simulink model "gps_casestudy_1_16"  (R2023a)
settings: Solver=VariableStepAuto  StartTime=0.0  StopTime=10.0  RelTol=1e-3
settings Model: PacingRate=0.890000  ExtModeTrigDuration=100  Creator=simon  LastModifiedBy=simon
settings DataIOCC: StateSaveName=tmp_raccel_xout  OutputSaveName=tmp_raccel_yout1  SignalLoggingName=tmp_raccel_logsout
settings OptimizationCC: EfficientMapNaN2IntZero=off  AccelVerboseBuild=on
settings HardwareCC: TargetBitPerPointer=64  TargetBitPerSizeT=64  TargetBitPerPtrDiffT=64  TargetLongLongMode=on  TargetIntDivRoundTo=Zero  TargetEndianess=LittleEndian  TargetWordSize=64  TargetHWDeviceType=MATLAB Host  ProdEqTarget=off
settings RTWCC: SystemTargetFile=raccel.tlc  TemplateMakefile=raccel_default_tmf  RTWVerbose=off  RTWUseSimCustomCode=on
settings CodeAppCC: GenerateComments=off  MaxIdLength=128  SimulinkBlockComments=off
settings RaccelTargetCC: TargetLangStandard=C99 (ISO)  OptimizeReductions=off  ENABLE_SLEXEC_SSBRIDGE=1  RTWCAPIParams=on  RTWCAPIRootIO=on

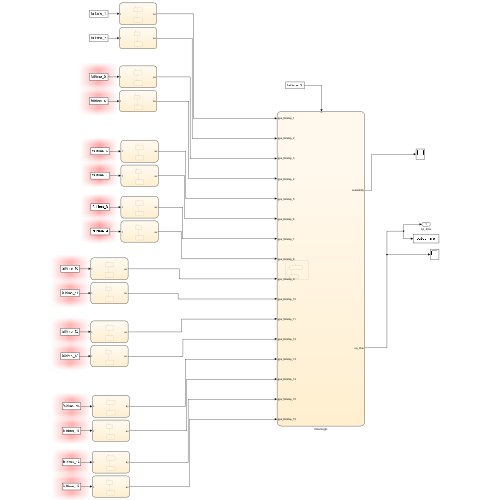
[thumbnail: Simulink's stored preview of the top-level diagram]
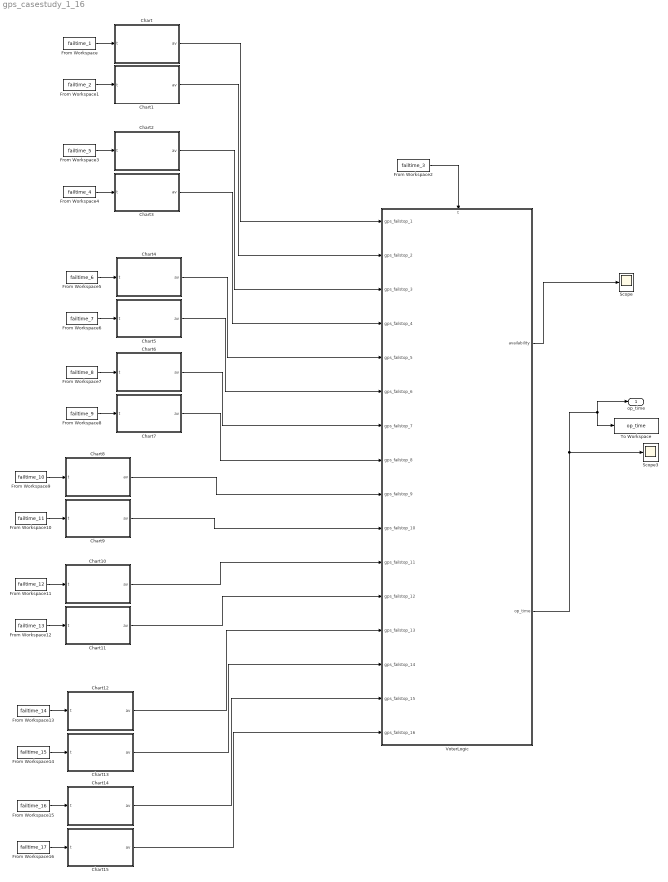
== system gps_casestudy_1_16 ==
  Chart : Stateflow chart  TreatAsAtomicUnit=on
  Chart1 : Stateflow chart  TreatAsAtomicUnit=on
  Chart10 : Stateflow chart  TreatAsAtomicUnit=on
  Chart11 : Stateflow chart  TreatAsAtomicUnit=on
  Chart12 : Stateflow chart  TreatAsAtomicUnit=on
  Chart13 : Stateflow chart  TreatAsAtomicUnit=on
  Chart14 : Stateflow chart  TreatAsAtomicUnit=on
  Chart15 : Stateflow chart  TreatAsAtomicUnit=on
  Chart2 : Stateflow chart  TreatAsAtomicUnit=on
  Chart3 : Stateflow chart  TreatAsAtomicUnit=on
  Chart4 : Stateflow chart  TreatAsAtomicUnit=on
  Chart5 : Stateflow chart  TreatAsAtomicUnit=on
  Chart6 : Stateflow chart  TreatAsAtomicUnit=on
  Chart7 : Stateflow chart  TreatAsAtomicUnit=on
  Chart8 : Stateflow chart  TreatAsAtomicUnit=on
  Chart9 : Stateflow chart  TreatAsAtomicUnit=on
  From Workspace : FromWorkspace  VariableName=failtime_1  SampleTime=-1
  From Workspace1 : FromWorkspace  VariableName=failtime_2  SampleTime=-1
  From Workspace10 : FromWorkspace  VariableName=failtime_11  SampleTime=-1
  From Workspace11 : FromWorkspace  VariableName=failtime_12  SampleTime=-1
  From Workspace12 : FromWorkspace  VariableName=failtime_13  SampleTime=-1
  From Workspace13 : FromWorkspace  VariableName=failtime_14  SampleTime=-1
  From Workspace14 : FromWorkspace  VariableName=failtime_15  SampleTime=-1
  From Workspace15 : FromWorkspace  VariableName=failtime_16  SampleTime=-1
  From Workspace16 : FromWorkspace  VariableName=failtime_17  SampleTime=-1
  From Workspace2 : FromWorkspace  VariableName=failtime_3  SampleTime=-1
  From Workspace3 : FromWorkspace  VariableName=failtime_5  SampleTime=-1
  From Workspace4 : FromWorkspace  VariableName=failtime_4  SampleTime=-1
  From Workspace5 : FromWorkspace  VariableName=failtime_6  SampleTime=-1
  From Workspace6 : FromWorkspace  VariableName=failtime_7  SampleTime=-1
  From Workspace7 : FromWorkspace  VariableName=failtime_8  SampleTime=-1
  From Workspace8 : FromWorkspace  VariableName=failtime_9  SampleTime=-1
  From Workspace9 : FromWorkspace  VariableName=failtime_10  SampleTime=-1
  Scope : Scope
  Scope3 : Scope
  To Workspace : ToWorkspace  VariableName=op_time  SaveFormat=Timeseries  SampleTime=-1
  VoterLogic : Stateflow chart  TreatAsAtomicUnit=on
      settings: PortSchema="{\"entries\":[{\"content\":{\"sides\":[{\"content\":{\"connectorIds\":[\"In1\",\"In2\",\"In3\",\"In4\",\"In5\",\"In6\",\"In7\",\"In8\",\"In9\",\"In10\",\"In11\",\"In12\",\"In13\",\"In15\",\"In14\",\"In16\"]},\"type\":\"ConnectorPlacement.EquallySpacedRectSide\",\"uuid\":\"b24c2d94-3c9d-4369-b965-d1338d6762d5\"},{\"content\":{\"connectorIds\":[\"Out1\",\"Out2\"],\"side\":\"RIGHT\"},\"type\":\"ConnectorPlacement.EquallySpacedRectSide\",\"uuid\":\"5f96e1c0-a37a-4ed1-9b99-6f6d53957bc9\"},{\"content\":{\"connectorIds\":[\"In17\"],\"side\":\"TOP\"},\"type\":\"ConnectorPlacement.EquallySpacedRectSide\",\"uuid\":\"3123bfe6-fcc6-4574-9210-ad2002987471\"}]},\"type\":\"ConnectorPlacement.EquallySpacedConnector\",\"uuid\":\"2f56b5a3-e193-4a43-bf0a-dc04d34b5817\"}],\"packageUris\":[\"http://schema.mathworks.com/mf0/Connector/R2020b\"],\"version\":\"1.0\"}"
  op_time : Outport
  wires:
  VoterLogic/1(availability) -> Scope/1
  VoterLogic/2(op_time) -> op_time/1, To Workspace/1, Scope3/1
  From Workspace1/1 -> Chart1/1(t)
  From Workspace/1 -> Chart/1(t)
  Chart/1(av) -> VoterLogic/1(gps_failstop_1)
  Chart1/1(av) -> VoterLogic/2(gps_failstop_2)
  From Workspace2/1 -> VoterLogic/17(t)
  Chart3/1(av) -> VoterLogic/4(gps_failstop_4)
  Chart2/1(av) -> VoterLogic/3(gps_failstop_3)
  From Workspace3/1 -> Chart2/1(t)
  From Workspace4/1 -> Chart3/1(t)
  From Workspace8/1 -> Chart7/1(t)
  From Workspace7/1 -> Chart6/1(t)
  Chart6/1(av) -> VoterLogic/7(gps_failstop_7)
  Chart7/1(av) -> VoterLogic/8(gps_failstop_8)
  Chart5/1(av) -> VoterLogic/6(gps_failstop_6)
  Chart4/1(av) -> VoterLogic/5(gps_failstop_5)
  From Workspace5/1 -> Chart4/1(t)
  From Workspace6/1 -> Chart5/1(t)
  From Workspace14/1 -> Chart13/1(t)
  From Workspace13/1 -> Chart12/1(t)
  Chart12/1(av) -> VoterLogic/13(gps_failstop_13)
  Chart13/1(av) -> VoterLogic/15(gps_failstop_14)
  Chart15/1(av) -> VoterLogic/16(gps_failstop_16)
  Chart14/1(av) -> VoterLogic/14(gps_failstop_15)
  From Workspace15/1 -> Chart14/1(t)
  From Workspace16/1 -> Chart15/1(t)
  From Workspace12/1 -> Chart11/1(t)
  From Workspace11/1 -> Chart10/1(t)
  Chart10/1(av) -> VoterLogic/11(gps_failstop_11)
  Chart11/1(av) -> VoterLogic/12(gps_failstop_12)
  Chart9/1(av) -> VoterLogic/10(gps_failstop_10)
  Chart8/1(av) -> VoterLogic/9(gps_failstop_9)
  From Workspace9/1 -> Chart8/1(t)
  From Workspace10/1 -> Chart9/1(t)

== stateflow chart gps_casestudy_1_16/Chart1 ==
  settings: updateMethod=CONTINUOUS
  state operational
    entry:
    av=1;
  state failstop
    entry:
    av=0;
  (default) -> operational
  operational -> failstop : after(t,sec)
  data: t input double; av output

== stateflow chart gps_casestudy_1_16/VoterLogic ==
  settings: updateMethod=CONTINUOUS  sampleTime=0.01  executeAtInitialization=1
  state reg2
    state Operation
      exit:
      op_time=temporalCount(sec)
    state Failstop
      entry: availability=0;
    (default) -> Operation : {availability=1}
    Operation -> Failstop [order 2] : after(t,sec)
    Operation -> Failstop [order 1] : [gps_failstop_1==0 && gps_failstop_2==0 && gps_failstop_3==0 && gps_failstop_4==0 && gps_failstop_5==0 && gps_failstop_6==0 && gps_failstop_7==0 && gps_failstop_8==0 && gps_failstop_9==0 && gps_failstop_10==0 && gps_failstop_11==0 && gps_failstop_12==0 && gps_failstop_13==0 && gps_failstop_14==0 && gps_failstop_15==0 && gps_failstop_16==0]
  (default) -> reg2
  data: availability output; op_time output double; gps_failstop_1 input; gps_failstop_2 input; gps_failstop_3 input; gps_failstop_4 input; gps_failstop_5 input; gps_failstop_6 input; gps_failstop_7 input; gps_failstop_8 input; gps_failstop_9 input; gps_failstop_10 input; gps_failstop_11 input; gps_failstop_12 input; gps_failstop_13 input; gps_failstop_15 input; gps_failstop_14 input; gps_failstop_16 input; t input

== stateflow chart gps_casestudy_1_16/Chart2 ==
  settings: updateMethod=CONTINUOUS
  state operational
    entry:
    av=1
  state failstop
    entry:
    av=0;
  (default) -> operational
  operational -> failstop : after(t,sec)
  data: t input double; av output

== stateflow chart gps_casestudy_1_16/Chart3 ==
  settings: updateMethod=CONTINUOUS
  state operational
    entry:
    av=1;
  state failstop
    entry:
    av=0;
  (default) -> operational
  operational -> failstop : after(t,sec)
  data: t input double; av output

== stateflow chart gps_casestudy_1_16/Chart4 ==
  settings: updateMethod=CONTINUOUS
  state operational
    entry:
    av=1
  state failstop
    entry:
    av=0;
  (default) -> operational
  operational -> failstop : after(t,sec)
  data: t input double; av output

== stateflow chart gps_casestudy_1_16/Chart5 ==
  settings: updateMethod=CONTINUOUS
  state operational
    entry:
    av=1;
  state failstop
    entry:
    av=0;
  (default) -> operational
  operational -> failstop : after(t,sec)
  data: t input double; av output

== stateflow chart gps_casestudy_1_16/Chart6 ==
  settings: updateMethod=CONTINUOUS
  state operational
    entry:
    av=1
  state failstop
    entry:
    av=0;
  (default) -> operational
  operational -> failstop : after(t,sec)
  data: t input double; av output

== stateflow chart gps_casestudy_1_16/Chart7 ==
  settings: updateMethod=CONTINUOUS
  state operational
    entry:
    av=1;
  state failstop
    entry:
    av=0;
  (default) -> operational
  operational -> failstop : after(t,sec)
  data: t input double; av output

== stateflow chart gps_casestudy_1_16/Chart10 ==
  settings: updateMethod=CONTINUOUS
  state operational
    entry:
    av=1
  state failstop
    entry:
    av=0;
  (default) -> operational
  operational -> failstop : after(t,sec)
  data: t input double; av output

== stateflow chart gps_casestudy_1_16/Chart11 ==
  settings: updateMethod=CONTINUOUS
  state operational
    entry:
    av=1;
  state failstop
    entry:
    av=0;
  (default) -> operational
  operational -> failstop : after(t,sec)
  data: t input double; av output

== stateflow chart gps_casestudy_1_16/Chart12 ==
  settings: updateMethod=CONTINUOUS
  state operational
    entry:
    av=1
  state failstop
    entry:
    av=0;
  (default) -> operational
  operational -> failstop : after(t,sec)
  data: t input double; av output

== stateflow chart gps_casestudy_1_16/Chart13 ==
  settings: updateMethod=CONTINUOUS
  state operational
    entry:
    av=1;
  state failstop
    entry:
    av=0;
  (default) -> operational
  operational -> failstop : after(t,sec)
  data: t input double; av output

== stateflow chart gps_casestudy_1_16/Chart14 ==
  settings: updateMethod=CONTINUOUS
  state operational
    entry:
    av=1
  state failstop
    entry:
    av=0;
  (default) -> operational
  operational -> failstop : after(t,sec)
  data: t input double; av output

== stateflow chart gps_casestudy_1_16/Chart15 ==
  settings: updateMethod=CONTINUOUS
  state operational
    entry:
    av=1;
  state failstop
    entry:
    av=0;
  (default) -> operational
  operational -> failstop : after(t,sec)
  data: t input double; av output

== stateflow chart gps_casestudy_1_16/Chart8 ==
  settings: updateMethod=CONTINUOUS
  state operational
    entry:
    av=1
  state failstop
    entry:
    av=0;
  (default) -> operational
  operational -> failstop : after(t,sec)
  data: t input double; av output

== stateflow chart gps_casestudy_1_16/Chart9 ==
  settings: updateMethod=CONTINUOUS
  state operational
    entry:
    av=1;
  state failstop
    entry:
    av=0;
  (default) -> operational
  operational -> failstop : after(t,sec)
  data: t input double; av output

== stateflow chart gps_casestudy_1_16/Chart ==
  settings: updateMethod=CONTINUOUS
  state operational
    entry:
    av=1
  state failstop
    entry:
    av=0;
  (default) -> operational
  operational -> failstop : after(t,sec)
  data: t input double; av output
